simulink model "learning_smc"  (R2020b)
settings: Solver=VariableStepAuto  StartTime=0.0  StopTime=30  RelTol=1e-3
settings Model: Creator=Taha  LastModifiedBy=Taha

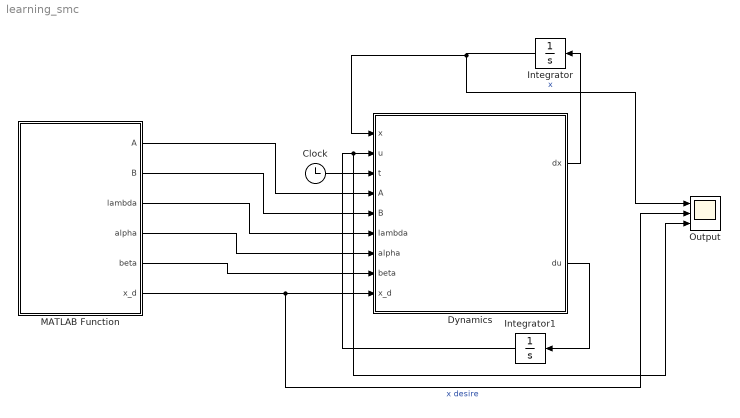
== system learning_smc ==
  Clock : Clock
  Dynamics : MATLAB Function  TreatAsAtomicUnit=on
  Integrator : Integrator  InitialCondition=0.05
  Integrator1 : Integrator  InitialCondition=0.01
  MATLAB Function : MATLAB Function  TreatAsAtomicUnit=on
  Output : Scope  NumInputPorts=3
  wires:
  Clock/1 -> Dynamics/3(t)
  Dynamics/2(du) -> Integrator1/1
  Dynamics/1(dx) -> Integrator/1
  Integrator/1 -> Dynamics/1(x), Output/1  "x"
  Integrator1/1 -> Output/3, Dynamics/2(u)
  MATLAB Function/1(A) -> Dynamics/4(A)
  MATLAB Function/2(B) -> Dynamics/5(B)
  MATLAB Function/3(lambda) -> Dynamics/6(lambda)
  MATLAB Function/4(alpha) -> Dynamics/7(alpha)
  MATLAB Function/5(beta) -> Dynamics/8(beta)
  MATLAB Function/6(x_d) -> Output/2, Dynamics/9(x_d)  "x desire"

== matlab function learning_smc/MATLAB Function ==
  data: A output; B output; lambda output; alpha output; beta output; x_d output
function [A,B,lambda,alpha,beta, x_d] = fcn()

A = 1;              % System matrix coefficient
B = 10;              % Control matrix coefficient
lambda = 80;       % Sliding surface coefficient
alpha = 40;          % Control coefficient
beta = 50;
x_d = 1;

== matlab function learning_smc/Dynamics ==
  data: x input; u input; dx output; t input; du output; A input; B input; lambda input; alpha input; beta input; x_d input
function [dx, du] = fcn(x,u, t, A,B, lambda,alpha,beta, x_d)

fx = 3 * x^2 + 2 * x^3;

dfx = 6 * x + 6 * x^2;

dt = 0.5 * sin(2 * t);

dx = A * x + B * u + fx + dt;


e = x - x_d;

de = dx;

s = de + lambda * e;


du = -1 * inv(B) * (A^2 * x + A*B*u + A*fx + dfx + lambda * A*x + ...
    lambda * B * u + lambda * fx + alpha * s + beta * sign(s));
